simulink model "PreisachContinuous"  (R2017b)
settings: Solver=FixedStepAuto  StartTime=0.0  StopTime=20.0  FixedStep=0.1  MaxStep=0.1  RelTol=1e-3
undefined symbols (not defined in the file): DiscIntNeverNeededParam, mu, muXMesh, muYMesh, shift, xLims, yLims
libraries: simulink x1
settings Model: Creator=M. Vasquez Beltran  LastModifiedBy=M. Vasquez Beltran

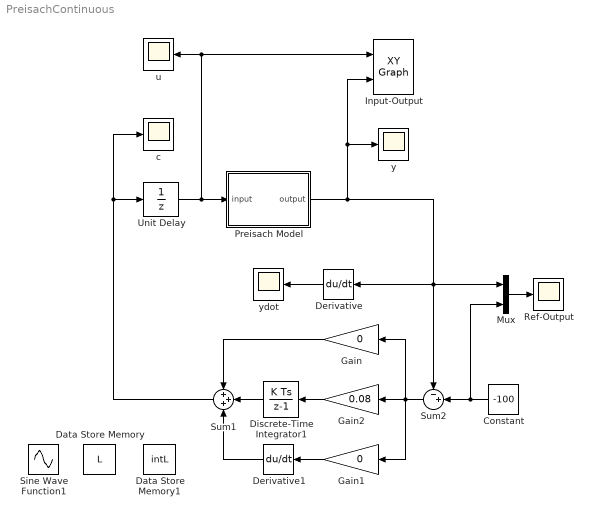
== system PreisachContinuous ==
  Constant : Constant  Value=-100
  Data Store Memory : DataStoreMemory  DataStoreName=L  ReadBeforeWriteMsg=warning  WriteAfterWriteMsg=warning  WriteAfterReadMsg=warning  ShowAdditionalParam=off  OutDataTypeStr=double  Dimensions=[500,2]
  Data Store Memory1 : DataStoreMemory  DataStoreName=intL  ReadBeforeWriteMsg=warning  WriteAfterWriteMsg=warning  WriteAfterReadMsg=warning  ShowAdditionalParam=off  OutDataTypeStr=double  Dimensions=[500,5]
  Derivative : Derivative  CoefficientInTFapproximation=10000
  Derivative1 : Derivative  CoefficientInTFapproximation=10000
  Discrete-Time Integrator1 : DiscreteIntegrator  gainval=1  InitialConditionSetting=State (most efficient)  SampleTime=-1  ICPrevOutput=DiscIntNeverNeededParam  ICPrevScaledInput=DiscIntNeverNeededParam
  Gain : Gain  Gain=0
  Gain1 : Gain  Gain=0
  Gain2 : Gain  Gain=0.08
  Input-Output : simulink/Sinks/XY Graph  xmin=-100*1.25  xmax=100*1.25  ymin=-3000*1.25  ymax=3000*1.25  st=-1
  Mux : Mux  Inputs=2
  Preisach Model : MATLAB Function  TreatAsAtomicUnit=on
  Ref-Output : Scope
  Sine Wave Function1 : Sin  Amplitude=100  Frequency=2*2*pi/20  Phase=90  SampleTime=0
  Sum1 : Sum  Inputs=+++
  Sum2 : Sum  Inputs=-+|
  Unit Delay : UnitDelay  SampleTime=-1
  c : Scope
  u : Scope
  y : Scope
  ydot : Scope
  wires:
  Mux/1 -> Ref-Output/1
  Sum2/1 -> Gain2/1, Gain1/1, Gain/1
  Preisach Model/1(output) -> Sum2/1, Derivative/1, Mux/1, Input-Output/2, y/1
  Unit Delay/1 -> Preisach Model/1(input), Input-Output/1, u/1
  Constant/1 -> Mux/2, Sum2/2
  Gain1/1 -> Derivative1/1
  Derivative/1 -> ydot/1
  Sum1/1 -> Unit Delay/1, c/1
  Gain2/1 -> Discrete-Time Integrator1/1
  Discrete-Time Integrator1/1 -> Sum1/2
  Gain/1 -> Sum1/1
  Derivative1/1 -> Sum1/3

== matlab function PreisachContinuous/Preisach Model ==
  settings: sampleTime=0.01
  data: input input; output output; mu parameter; muXMesh parameter; muYMesh parameter; xLims parameter; yLims parameter; shift parameter; L data_store_memory size=[500 2]; intL data_store_memory size=[500 5]
function output  = fcn(input, mu, muXMesh, muYMesh, xLims, yLims, shift)

output = 0;

L = varL();
intL = varIntL();

L = updateL(L, input, xLims, yLims);
[output, intL] = computeInterpOutput(L, intL, mu, muXMesh, muYMesh, xLims, yLims);
output = output + shift;

varL(L);
varIntL(intL);

end

function L = updateL(L, u, xLims, yLims)
    if(u>xLims(2) || u>yLims(2))
        u = min(xLims(2), yLims(2));
    elseif(u<xLims(1) || u<yLims(1))
        u = max(xLims(1), yLims(1));
    end
    if(size(L,1)<1 || size(L,2)~=2)
        L = [xLims(1), yLims(2); 
            xLims(1), u; 
            u,u];
    end
    i = 2;
    while(i<size(L,1))
        if( (L(i-1,1)==L(i,1) && L(i,1)==L(i+1,1))...
            || (L(i-1,2)==L(i,2) && L(i,2)==L(i+1,2)) )
            L(i,:) = [];
        else
            i = i+1;
        end
    end
    for i=1:size(L,1)
        if((L(i,1)<=u && L(i,2)>u) || (L(i,1)<u && L(i,2)>=u))
            continue;
        elseif (L(i,1)>u && L(i,2)>u)
            L = [L(1:i-1,:); u, L(i,2); u,u];
            break;
        elseif (L(i,1)<u && L(i,2)<u)
            L = [L(1:i-1,:); L(i,1), u; u,u];
            break;
        else
            L = [L(1:i-1,:); u,u];
            break;
        end
    end
end

function [output, intL] = computeInterpOutput(L, intL, mu, muXMesh, muYMesh, xLims, yLims)
    output = 0;
    
    if(size(intL,1)<1 || size(intL,2)~=5)
        intL = zeros(1,5);
    end
    
    if(size(L,1)<2)
        return;
    end
    
    for i=1:size(L,1)-1
        if(L(i,2)==L(i+1,2))
            if( size(intL,1)>=i && isequal(intL(i,1:4), [L(i,1), L(i+1,1), L(i,2), yLims(2)]) )
                output = output + intL(i,5);
            else
                integralVal = integralInterp(muXMesh, muYMesh, mu, [L(i,1), L(i+1,1)], [L(i,2), yLims(2)]);
                intL = [intL; L(i,1), L(i+1,1), L(i,2), yLims(2), integralVal];
                output = output + integralVal;
            end
        elseif(L(i,1)==L(i+1,1))
            if( size(intL,1)>=i && isequal(intL(i,1:4), [xLims(1), L(i,1), L(i+1,2), L(i,2)]) )
                output = output - intL(i,5);
            else
                integralVal = integralInterp(muXMesh, muYMesh, mu, [xLims(1), L(i,1)], [L(i+1,2), L(i,2)]);
                intL = [intL; xLims(1), L(i,1), L(i+1,2), L(i,2), integralVal]; 
                output = output - integralVal;
            end
        end 
    end
    if (size(intL,1)>=i+1 && isequal(intL(i+1,1:4), [xLims(1), L(end,1), yLims(1), L(end,2)]) )
        output = output + intL(i+1,5);
    else
        integralVal = integralInterp(muXMesh, muYMesh, mu, [xLims(1), L(end,1)], [yLims(1), L(end,2)]);
        intL = [intL; xLims(1), L(end,1), yLims(1), L(end,2), integralVal];
        output = output + integralVal;
    end
    if (size(intL,1)>=i+2 && isequal(intL(i+2,1:4), [L(end,1), xLims(2), L(end,2), yLims(2)]) )
        output = output - intL(i+2,5);
    else
        integralVal = integralInterp(muXMesh, muYMesh, mu, [L(end,1), xLims(2)], [L(end,2), yLims(2)]);
        intL = [intL; L(end,1), xLims(2), L(end,2), yLims(2), integralVal];
        output = output - integralVal;
    end
    intL = intL(1:i+2,:);
    
%     output = output...
%         - integral2(@maskSimpleMu, intL(end,1), xLims(2), intL(end,2), yLims(2))...
%         + integral2(@maskSimpleMu, xLims(1), intL(end,1), yLims(1), intL(end,2));  
%     for i=2:size(intL,1)
%         if(intL(i,2)==intL(i+1,2))
%             output = output...
%                 + integral2(@maskSimpleMu, intL(i,1), intL(i+1,1), intL(i,2), yLims(2));
%         elseif(intL(i,1)==intL(i+1,1))
%             output = output...
%                 - integral2(@maskSimpleMu, xLims(1), intL(i+1,1), intL(i+1,2), intL(i,2));
%         end 
%     end
end

function val = integralInterp(muXMesh, muYMesh, mu, xLims, yLims)
%     interpXN = max([600, min([100, ceil(abs(xLims(2)-xLims(1)))/0.1])]);
%     interpYN = max([300, min([100, ceil(abs(yLims(2)-yLims(1)))/10])]);
    interpXN = 200;
    interpYN = 200;
    xDiff = (xLims(2)-xLims(1))/(interpXN-1);
    yDiff = (yLims(2)-yLims(1))/(interpYN-1);
    xInterpGrid = linspace(xLims(1), xLims(2), interpXN);
    yInterpGrid = linspace(yLims(1), yLims(2), interpYN);
    [xInterpMesh, yInterpMesh] = meshgrid(xInterpGrid, yInterpGrid);
    
    interpMu = interp2(muXMesh, muYMesh, mu, xInterpMesh, yInterpMesh, 'spline');
    interpMu(isnan(interpMu)) = 0;
    
    val = sum(sum(interpMu.*(xDiff*yDiff)));
end

function y = varL(varargin)
    persistent L;
    if isempty(L)
        coder.varsize('L',[1000,2], [1,0]);
        L = zeros(0,2);
    end
    if nargin > 0
        L = [varargin{1}];
    end
    y = L;
end

function y = varIntL(varargin)
    persistent intL;
    if isempty(intL)
        coder.varsize('intL',[1000,5], [1,0]);
        intL = zeros(0,5);
    end
    if nargin > 0
        intL = [varargin{1}];
    end
    y = intL;
end
